simulink model "machine_bloc"  (R2019b)
settings: Solver=VariableStepAuto  StartTime=0.0  StopTime=2  RelTol=1e-3
libraries: powerlib x6, simulink x1
settings Model: Creator=x1 yoga  LastModifiedBy=x1 yoga

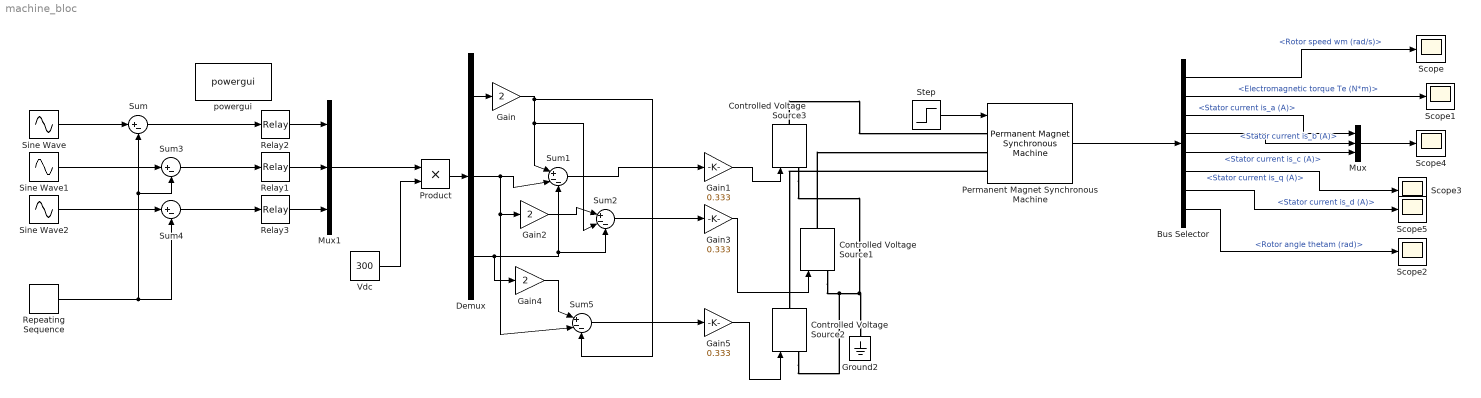
== system machine_bloc ==
  Bus Selector : BusSelector  OutputSignals=Rotor speed wm (rad/s),Electromagnetic torque Te (N*m),Stator current is_a (A),Stator current is_b (A),Stator current is_c (A),Stator current is_q (A),Stator current is_d (A),Rotor angle thetam (rad)
  Controlled Voltage Source1 : powerlib/Electrical Sources/Controlled Voltage Source  Initialize=on  Source_Type=AC  Amplitude=0  Phase=0  Frequency=0  Measurements=None
      settings: SourceProductName=Simscape Electrical
  Controlled Voltage Source2 : powerlib/Electrical Sources/Controlled Voltage Source  Initialize=on  Source_Type=AC  Amplitude=0  Phase=0  Frequency=0  Measurements=None
      settings: SourceProductName=Simscape Electrical
  Controlled Voltage Source3 : powerlib/Electrical Sources/Controlled Voltage Source  Initialize=on  Source_Type=AC  Amplitude=0  Phase=0  Frequency=0  Measurements=None
      settings: SourceProductName=Simscape Electrical
  Demux : Demux  Outputs=3
  Gain : Gain  Gain=2
  Gain1 : Gain  Gain=0.333
  Gain2 : Gain  Gain=2
  Gain3 : Gain  Gain=0.333
  Gain4 : Gain  Gain=2
  Gain5 : Gain  Gain=0.333
  Ground2 : powerlib/Elements/Ground  LConnTagsString=a
      settings: SourceProductName=Simscape Electrical
  Mux : Mux  Inputs=3
  Mux1 : Mux  Inputs=3
  Permanent Magnet Synchronous Machine : powerlib/Machines/Permanent Magnet Synchronous Machine  NbPhases=3  FluxDistribution=Sinusoidal  RotorType=Salient-pole  MechanicalLoad=Torque Tm  PresetModel=No  ShowDetailedParameters=on  MeasurementBus=off  Resistance=0.8  Inductance=8.5e-3  dqInductances=[1.10e-3 1.32e-3]  La=0.000395  MachineConstant=Flux linkage established by magnets (V.s)  Flux=0.15  VoltageCst=54.414  TorqueCst=0.45  Flat=120  Mechanical=[1.15e-3 0.59e-4 2 0]  PolePairs=4  InitialConditions=[0,0, 0,0]  InitialConditions5ph=[0 0 0 0 0 0]  RefAngle=Aligned with phase A axis (original Park)  IterativeDiscreteModel=Trapezoidal non iterative  TsBlock=-1  TsPowergui=0
  Product : Product
  Relay1 : Relay  OnSwitchValue=0.1  OffSwitchValue=-0.1  OffOutputValue=-1
  Relay2 : Relay  OnSwitchValue=0.1  OffSwitchValue=-0.1  OffOutputValue=-1
  Relay3 : Relay  OnSwitchValue=0.1  OffSwitchValue=-0.1  OffOutputValue=-1
  Repeating Sequence : simulink/Sources/Repeating Sequence  rep_seq_t=[0 0.00025 0.0005]  rep_seq_y=[0 1 0]
  Scope{,1..5} (6 alike) : Scope
  Sine Wave : Sin  Amplitude=100  Frequency=2*pi*50  SampleTime=0
  Sine Wave1 : Sin  Amplitude=100  Frequency=2*pi*50  Phase=-2*pi/3  SampleTime=0
  Sine Wave2 : Sin  Amplitude=100  Frequency=2*pi*50  Phase=2*pi/3  SampleTime=0
  Step : Step  Time=1.2  After=23  SampleTime=0
  Sum : Sum  Inputs=|+-
  Sum1 : Sum  Inputs=|+--
  Sum2 : Sum  Inputs=|+--
  Sum3 : Sum  Inputs=|+-
  Sum4 : Sum  Inputs=|+-
  Sum5 : Sum  Inputs=|+--
  "Vdc " : Constant  Value=300
  powergui : powerlib/powergui  Priority=1  SimulationMode=Continuous  SampleTime=50e-6  frequency=60  Iterations=50  frequencyindice=0  Pbase=100e6  ErrMax=1e-4  UnitsV=kV  UnitsW=MW  buscounter=0  FunctionMessages=off  echomessages=off  EnableUseOfTLC=off  CurrentSourceSwitches=off  DisableSnubberDevices=off  DisableRonSwitches=off  DisableVfSwitches=off  DisplayEquations=off  AutomaticDiscreteSolvers=off  SolverType=Tustin/Backward Euler (TBE)  Interpol=off  ExternalGateDelay=off  methode=off  Ts=100  x0status=blocks  SPID=on  SwTol=0  HookPort=off  NonlinearTolerance=1e-4  nMaxIteration=100  ContinueOnMaxIteration=off  RestoreLinks=warning  ResistiveCurrentMeasurement=off  Frange=[0:2:500]  Ylog=off  Xlog=on  ShowGrid=off  save=off  variable=ZData  structure=0  ZoomFFT=off  StartTime=0.0  cycles=1  DisplayStyle=1  fundamental=60  FreqAxis=off  MaxFrequency=1000  frequencyindicesteady=1  RmsSteady=1  display=off
      settings: SourceProductName=Simscape Electrical
  wires:
  Bus Selector/1 -> Scope/1  "<Rotor speed wm (rad/s)>"
  Bus Selector/2 -> Scope1/1  "<Electromagnetic torque Te (N*m)>"
  Bus Selector/3 -> Mux/1  "<Stator current is_a (A)>"
  Bus Selector/4 -> Mux/2  "<Stator current is_b (A)>"
  Bus Selector/5 -> Mux/3  "<Stator current is_c (A)>"
  Mux/1 -> Scope4/1
  Bus Selector/6 -> Scope3/1  "<Stator current is_q (A)>"
  Bus Selector/7 -> Scope5/1  "<Stator current is_d (A)>"
  Bus Selector/8 -> Scope2/1  "<Rotor angle thetam (rad)>"
  Step/1 -> Permanent Magnet Synchronous Machine/1
  Permanent Magnet Synchronous Machine/1 -> Bus Selector/1
  Product/1 -> Demux/1
  Sine Wave/1 -> Sum/1
  Sum3/1 -> Relay1/1
  Sum4/1 -> Relay3/1
  Sine Wave1/1 -> Sum3/1
  Sine Wave2/1 -> Sum4/1
  Sum/1 -> Relay2/1
  Gain/1 -> Sum5/3, Sum2/2, Sum1/1
  Demux/2 -> Sum5/2, Gain2/1, Sum1/2
  Repeating Sequence/1 -> Sum3/2, Sum/2, Sum4/2
  Relay1/1 -> Mux1/2
  Demux/1 -> Gain/1
  "Vdc "/1 -> Product/2
  Sum1/1 -> Gain1/1
  Relay2/1 -> Mux1/1
  Mux1/1 -> Product/1
  Relay3/1 -> Mux1/3
  Demux/3 -> Gain4/1, Sum2/3, Sum1/3
  Gain2/1 -> Sum2/1
  Sum2/1 -> Gain3/1
  Gain4/1 -> Sum5/1
  Sum5/1 -> Gain5/1
  Gain3/1 -> Controlled Voltage Source1/1
  Gain5/1 -> Controlled Voltage Source2/1
  Gain1/1 -> Controlled Voltage Source3/1
  connections:
  Controlled Voltage Source3/RConn1 -- Permanent Magnet Synchronous Machine/LConn1
  Controlled Voltage Source1/LConn1 -- Controlled Voltage Source2/LConn1 -- Controlled Voltage Source3/LConn1 -- Ground2/LConn1
  Permanent Magnet Synchronous Machine/LConn3 -- Controlled Voltage Source2/RConn1
  Controlled Voltage Source1/RConn1 -- Permanent Magnet Synchronous Machine/LConn2
